simulink model "fuzzypi_bldc"  (R2024a)
settings: Solver=VariableStepAuto  StartTime=0.0  StopTime=10  RelTol=1e-3
undefined symbols (not defined in the file): ts
libraries: simulink x6, spsVoltageMeasurementLib x2, spsControlledVoltageSourceLib x1, spsPermanentMagnetSynchronousMachineLib x1, fuzblock x1, spsUniversalBridgeLib x1, sps_lib x1
settings Model: Creator=HP  LastModifiedBy=HP

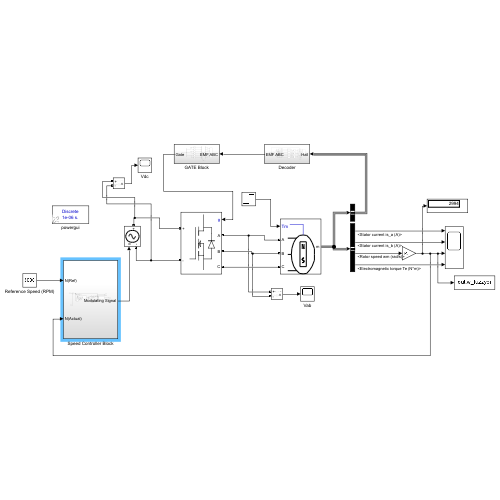
[thumbnail: Simulink's stored preview of the top-level diagram]
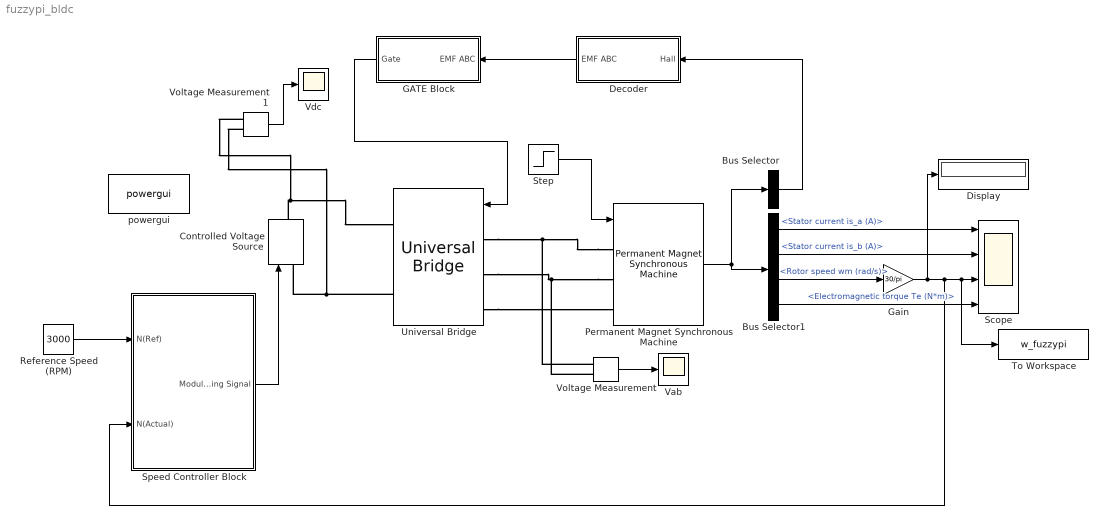
== system fuzzypi_bldc ==
  Bus Selector : BusSelector  OutputSignals=Hall effect signal h_a,Hall effect signal h_b,Hall effect signal h_c  OutputAsBus=on
  Bus Selector1 : BusSelector  OutputSignals=Stator current is_a (A),Stator current is_b (A),Rotor speed wm (rad/s),Electromagnetic torque Te (N*m)
  Controlled Voltage Source : spsControlledVoltageSourceLib/Controlled Voltage Source  Initialize=on  Source_Type=AC  Amplitude=0  Phase=0  Frequency=0  Measurements=None
  Decoder : Subsystem
  Display : Display
  GATE Block : Subsystem
  Gain : Gain  Gain=30/pi
  Permanent Magnet Synchronous Machine : spsPermanentMagnetSynchronousMachineLib/Permanent Magnet Synchronous Machine  NbPhases=3  FluxDistribution=Trapezoidal  RotorType=Round  MechanicalLoad=Torque Tm  PresetModel=No  ShowDetailedParameters=on  MeasurementBus=off  Resistance=0.0485  Inductance=8.5e-3  dqInductances=[8.5e-3,8.5e-3]  La=0.000395  MachineConstant=Flux linkage established by magnets (V.s)  Flux=0.1194  VoltageCst=100.0283  TorqueCst=0.9552  Flat=120  Mechanical=[0.0027 0.0004924 4 0]  PolePairs=4  InitialConditions=[0,0, 0,0]  InitialConditions5ph=[0 0 0 0 0 0]  RefAngle=90 degrees behind phase A axis (modified Park)  IterativeDiscreteModel=Trapezoidal non iterative  TsBlock=-1  TsPowergui=0
  Reference Speed (RPM) : Constant  Value=3000
  Scope : Scope  NumInputPorts=4
  Speed Controller Block : Subsystem
  Step : Step  Time=.1  After=3  SampleTime=0
  To Workspace : ToWorkspace  VariableName=w_fuzzypi  SampleTime=-1
  Universal Bridge : spsUniversalBridgeLib/Universal Bridge  Arms=3  SnubberResistance=1e5  SnubberCapacitance=inf  Device=MOSFET / Diodes  Ron=1e-3  Lon=0  ForwardVoltages="[  0  0  ]"  ForwardVoltage=0  GTOparameters=[ 10e-6 , 20e-6 ]  IGBTparameters=[ 1e-6 , 2e-6 ]  Measurements=None  Measurements_2=None  converterType=Rectifier
  Vab : Scope
  Vdc : Scope
  Voltage Measurement : spsVoltageMeasurementLib/Voltage Measurement  PhasorSimulation=off  OutputType=Complex  PSBequivalent=0
  Voltage Measurement1 : spsVoltageMeasurementLib/Voltage Measurement  PhasorSimulation=off  OutputType=Complex  PSBequivalent=0
  powergui : sps_lib/powergui  Priority=1  SimulationMode=Discrete  SampleTime=ts  frequency=60  Iterations=50  frequencyindice=0  Pbase=100e6  ErrMax=1e-4  UnitsV=kV  UnitsW=MW  buscounter=0  FunctionMessages=off  echomessages=off  EnableUseOfTLC=off  CurrentSourceSwitches=off  DisableSnubberDevices=off  DisableRonSwitches=off  DisableVfSwitches=off  DisplayEquations=off  AutomaticDiscreteSolvers=off  SolverType=Tustin/Backward Euler (TBE)  Interpol=off  ExternalGateDelay=off  methode=off  Ts=100  x0status=blocks  SPID=on  SwTol=0  HookPort=off  NonlinearTolerance=1e-4  nMaxIteration=100  ContinueOnMaxIteration=off  RestoreLinks=warning  ResistiveCurrentMeasurement=off  Frange=[0:2:500]  Ylog=off  Xlog=on  ShowGrid=off  save=off  variable=ZData  structure=0  ZoomFFT=off  StartTime=0.0  cycles=1  DisplayStyle=1  fundamental=60  FreqAxis=off  MaxFrequency=1000  frequencyindicesteady=1  RmsSteady=1  display=off
  wires:
  Bus Selector1/4 -> Scope/4  "<Electromagnetic torque Te (N*m)>"
  Gain/1 -> Display/1, Speed Controller Block/2(N(Actual)), To Workspace/1, Scope/3
  Decoder/1(EMF ABC) -> GATE Block/1(EMF ABC)
  Bus Selector/1 -> Decoder/1(Hall)
  GATE Block/1(Gate) -> Universal Bridge/1
  Step/1 -> Permanent Magnet Synchronous Machine/1
  Voltage Measurement/1 -> Vab/1
  Bus Selector1/3 -> Gain/1  "<Rotor speed wm (rad/s)>"
  Permanent Magnet Synchronous Machine/1 -> Bus Selector1/1, Bus Selector/1
  Bus Selector1/1 -> Scope/1  "<Stator current is_a (A)>"
  Bus Selector1/2 -> Scope/2  "<Stator current is_b (A)>"
  Voltage Measurement1/1 -> Vdc/1
  Speed Controller Block/1(Modulating Signal) -> Controlled Voltage Source/1
  Reference Speed (RPM)/1 -> Speed Controller Block/1(N(Ref))
  connections:
  Permanent Magnet Synchronous Machine/LConn2 -- Universal Bridge/LConn2 -- Voltage Measurement/LConn2
  Permanent Magnet Synchronous Machine/LConn1 -- Universal Bridge/LConn1 -- Voltage Measurement/LConn1
  Universal Bridge/RConn2 -- Voltage Measurement1/LConn2 -- Controlled Voltage Source/LConn1
  Universal Bridge/LConn3 -- Permanent Magnet Synchronous Machine/LConn3
  Controlled Voltage Source/RConn1 -- Voltage Measurement1/LConn1 -- Universal Bridge/RConn1

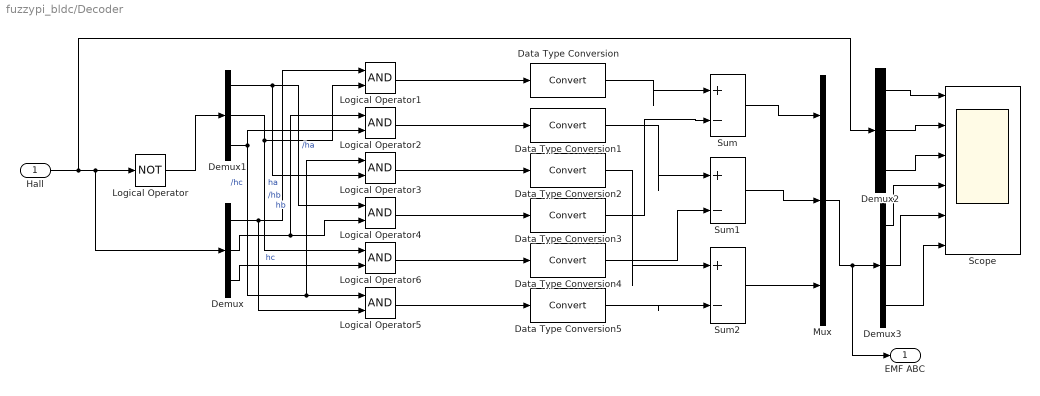
== system fuzzypi_bldc/Decoder ==
  Hall : Inport
  Data Type Conversion{,1..5} (6 alike) : DataTypeConversion  SaturateOnIntegerOverflow=off  RndMeth=Floor
  Demux{,1..3} (4 alike) : Demux  Outputs=3
  Logical Operator : Logic  Operator=NOT  AllPortsSameDT=off  OutDataTypeStr=boolean
  Logical Operator{1..6} (6 alike) : Logic  AllPortsSameDT=off  OutDataTypeStr=boolean
  Mux : Mux  Inputs=3
  Scope : Scope  NumInputPorts=6
  Sum : Sum  Inputs=|+-
  Sum1 : Sum  Inputs=|+-
  Sum2 : Sum  Inputs=|+-
  EMF ABC : Outport
  wires:
  Hall/1 -> Demux2/1, Demux/1, Logical Operator/1
  Logical Operator/1 -> Demux1/1
  Logical Operator1/1 -> Data Type Conversion/1
  Logical Operator2/1 -> Data Type Conversion1/1
  Logical Operator3/1 -> Data Type Conversion2/1
  Logical Operator4/1 -> Data Type Conversion3/1
  Logical Operator6/1 -> Data Type Conversion4/1
  Logical Operator5/1 -> Data Type Conversion5/1
  Data Type Conversion/1 -> Sum/1
  Data Type Conversion1/1 -> Sum1/1
  Data Type Conversion2/1 -> Sum2/1
  Data Type Conversion3/1 -> Sum/2
  Data Type Conversion4/1 -> Sum1/2
  Data Type Conversion5/1 -> Sum2/2
  Sum/1 -> Mux/1
  Sum1/1 -> Mux/2
  Sum2/1 -> Mux/3
  Mux/1 -> EMF ABC/1, Demux3/1
  Demux2/1 -> Scope/1
  Demux2/2 -> Scope/2
  Demux2/3 -> Scope/3
  Demux3/1 -> Scope/4
  Demux3/2 -> Scope/5
  Demux3/3 -> Scope/6
  Demux1/1 -> Logical Operator3/2, Logical Operator4/1  "/ha"
  Demux1/2 -> Logical Operator1/2, Logical Operator6/1  "/hb"
  Demux1/3 -> Logical Operator3/1, Logical Operator5/1, Logical Operator2/2  "/hc"
  Demux/1 -> Logical Operator5/2, Logical Operator1/1  "ha"
  Demux/2 -> Logical Operator2/1, Logical Operator4/2  "hb"
  Demux/3 -> Logical Operator6/2  "hc"

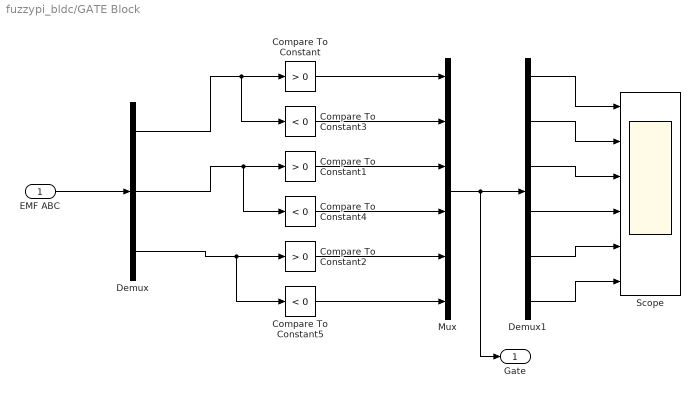
== system fuzzypi_bldc/GATE Block ==
  EMF ABC : Inport
  Compare To Constant : simulink/Logic and Bit Operations/Compare To Constant  relop=>  const=0  OutDataTypeStr=boolean
  Compare To Constant1 : simulink/Logic and Bit Operations/Compare To Constant  relop=>  const=0  OutDataTypeStr=boolean
  Compare To Constant2 : simulink/Logic and Bit Operations/Compare To Constant  relop=>  const=0  OutDataTypeStr=boolean
  Compare To Constant3 : simulink/Logic and Bit Operations/Compare To Constant  relop=<  const=0  OutDataTypeStr=boolean
  Compare To Constant4 : simulink/Logic and Bit Operations/Compare To Constant  relop=<  const=0  OutDataTypeStr=boolean
  Compare To Constant5 : simulink/Logic and Bit Operations/Compare To Constant  relop=<  const=0  OutDataTypeStr=boolean
  Demux : Demux  Outputs=3
  Demux1 : Demux  Outputs=6
  Mux : Mux  Inputs=6
  Scope : Scope  NumInputPorts=6
  Gate : Outport
  wires:
  EMF ABC/1 -> Demux/1
  Demux/1 -> Compare To Constant3/1, Compare To Constant/1
  Demux/2 -> Compare To Constant4/1, Compare To Constant1/1
  Demux/3 -> Compare To Constant5/1, Compare To Constant2/1
  Compare To Constant/1 -> Mux/1
  Compare To Constant3/1 -> Mux/2
  Compare To Constant1/1 -> Mux/3
  Compare To Constant4/1 -> Mux/4
  Compare To Constant2/1 -> Mux/5
  Compare To Constant5/1 -> Mux/6
  Mux/1 -> Gate/1, Demux1/1
  Demux1/1 -> Scope/1
  Demux1/2 -> Scope/2
  Demux1/3 -> Scope/3
  Demux1/4 -> Scope/4
  Demux1/5 -> Scope/5
  Demux1/6 -> Scope/6

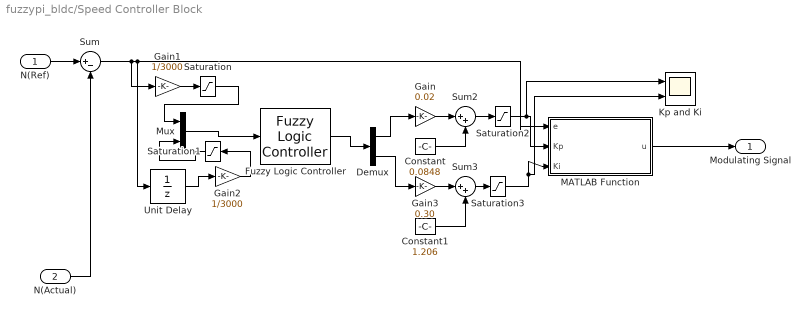
== system fuzzypi_bldc/Speed Controller Block ==
  N(Ref) : Inport
  N(Actual) : Inport  Port=2
  Constant : Constant  Value=0.0848
  Constant1 : Constant  Value=1.206
  Demux : Demux  Outputs=2
  Fuzzy Logic Controller : fuzblock/Fuzzy Logic  Controller  FIS=fuzzypi  OutputSampleNumber=101  DataType=double  FuzzifiedInputs=off  RuleFiringStrengths=off  RuleOutputs=off  AggregatedOutputs=off  SimulateUsing=Interpreted execution  OutOfRangeInputValueMessage=warning  NoRuleFiredMessage=warning  EmptyOutputFuzzySetMessage=warning
  Gain : Gain  Gain=0.02
  Gain1 : Gain  Gain=1/3000
  Gain2 : Gain  Gain=1/3000
  Gain3 : Gain  Gain=0.30
  Kp and Ki : Scope  NumInputPorts=2
  MATLAB Function : MATLAB Function  TreatAsAtomicUnit=on
  Mux : Mux  Inputs=2
  Saturation : Saturate  UpperLimit=1  LowerLimit=-1
  Saturation1 : Saturate  UpperLimit=1  LowerLimit=-1
  Saturation2 : Saturate  UpperLimit=0.13  LowerLimit=0.04
  Saturation3 : Saturate  UpperLimit=1.8  LowerLimit=0.6
  Sum : Sum  Inputs=|+-
  Sum2 : Sum  Inputs=|++
  Sum3 : Sum  Inputs=|++
  Unit Delay : UnitDelay  SampleTime=-1  HasFrameUpgradeWarning=on
  Modulating Signal : Outport
  wires:
  N(Ref)/1 -> Sum/1
  Sum/1 -> MATLAB Function/1(e), Unit Delay/1, Gain1/1
  Mux/1 -> Fuzzy Logic Controller/1
  Fuzzy Logic Controller/1 -> Demux/1
  Demux/1 -> Gain/1
  MATLAB Function/1(u) -> Modulating Signal/1
  Unit Delay/1 -> Gain2/1
  N(Actual)/1 -> Sum/2
  Gain1/1 -> Saturation/1
  Saturation/1 -> Mux/1
  Gain2/1 -> Saturation1/1
  Saturation1/1 -> Mux/2
  Demux/2 -> Gain3/1
  Gain/1 -> Sum2/1
  Constant/1 -> Sum2/2
  Gain3/1 -> Sum3/1
  Constant1/1 -> Sum3/2
  Sum2/1 -> Saturation2/1
  Sum3/1 -> Saturation3/1
  Saturation2/1 -> Kp and Ki/1, MATLAB Function/2(Kp)
  Saturation3/1 -> Kp and Ki/2, MATLAB Function/3(Ki)

== matlab function fuzzypi_bldc/Speed Controller Block/MATLAB Function ==
  data: e input; u output; Kp input; Ki input
function u = Adaptive_PI(e,Kp,Ki)
%#codegen

persistent integral

if isempty(integral)
    integral = 0;
end

Ts = 1e-6;

integral = integral + e*Ts;

u = Kp*e + Ki*integral;

end
